simulink model "yixiang"  (R2024a)
settings: Solver=FixedStepDiscrete  StartTime=0.0  StopTime=0.01  FixedStep=1e-8  RelTol=1e-3
libraries: hdlsllib x60, simulink x1
(part 2 of 2)

== system yixiang/CBSVPWM/jxcbsv/yixianga ==
  aH1 : Inport
  zmc1 : Subsystem
  zmcxc6 : Subsystem
  aHyan : Outport
  wires:
  zmcxc6/1(aL1) -> aHyan/1
  zmc1/1(bH1) -> zmcxc6/1(bH1)
  aH1/1 -> zmc1/1(aH1)

== system yixiang/CBSVPWM/jxcbsv/zmc ==
  aH1 : Inport
  Constant2 : Constant  OutDataTypeStr=int16  SampleTime=2E-8
  Constant3 : Constant  Commented=on  Value=0  OutDataTypeStr=int16  SampleTime=2e-8
  Data Type Conversion1 : DataTypeConversion  OutDataTypeStr=boolean  SaturateOnIntegerOverflow=off  RndMeth=Floor
  Data Type Conversion2 : DataTypeConversion  OutDataTypeStr=boolean  SaturateOnIntegerOverflow=off  RndMeth=Floor
  Data Type Conversion3 : DataTypeConversion  Commented=on  OutDataTypeStr=boolean  SaturateOnIntegerOverflow=off  RndMeth=Floor
  HDL Counter1 : hdlsllib/Sources/HDL Counter  Commented=on  CountType=Free running  CountInit=0  CountStep=1  CountMax=250  CountFromType=Initial value  CountFrom=0  CountResetPort=on  CountLoadPort=off  CountEnbPort=off  CountDirPort=off  CountHitOutputPort=off  CountDataType=Signed  CountWordLen=16  CountFracLen=0  CountSampTime=2E-8
  HDL Counter7 : hdlsllib/Sources/HDL Counter  CountType=Free running  CountInit=0  CountStep=1  CountMax=250  CountFromType=Initial value  CountFrom=0  CountResetPort=on  CountLoadPort=off  CountEnbPort=on  CountDirPort=off  CountHitOutputPort=off  CountDataType=Signed  CountWordLen=16  CountFracLen=0  CountSampTime=1
  Logical Operator : Logic  Operator=NOT  AllPortsSameDT=off  OutDataTypeStr=boolean
  Logical Operator1 : Logic  Commented=on  Operator=NOT  AllPortsSameDT=off  OutDataTypeStr=boolean
  Scope6 : Scope  NumInputPorts=2
  Switch : Switch  Threshold=3  SaturateOnIntegerOverflow=off  InputSameDT=off
  Switch2 : Switch  Commented=on  Threshold=1  SaturateOnIntegerOverflow=off  InputSameDT=off
  bH1 : Outport
  wires:
  HDL Counter7/1 -> Switch/2, Scope6/1
  Data Type Conversion1/1 -> Logical Operator/1
  Constant2/1 -> Switch/3
  aH1/1 -> Data Type Conversion1/1, Scope6/2, Data Type Conversion2/1, Switch/1
  Logical Operator/1 -> HDL Counter7/2
  Data Type Conversion2/1 -> HDL Counter7/1
  Constant3/1 -> Switch2/3
  HDL Counter1/1 -> Switch2/2
  Switch/1 -> bH1/1
  Data Type Conversion3/1 -> Logical Operator1/1
  Logical Operator1/1 -> HDL Counter1/1

== system yixiang/CBSVPWM/jxcbsv/zmc1 ==
  aH1 : Inport
  Constant2 : Constant  OutDataTypeStr=int16  SampleTime=2E-8
  Constant3 : Constant  Commented=on  Value=0  OutDataTypeStr=int16  SampleTime=2e-8
  Data Type Conversion1 : DataTypeConversion  OutDataTypeStr=boolean  SaturateOnIntegerOverflow=off  RndMeth=Floor
  Data Type Conversion2 : DataTypeConversion  OutDataTypeStr=boolean  SaturateOnIntegerOverflow=off  RndMeth=Floor
  Data Type Conversion3 : DataTypeConversion  Commented=on  OutDataTypeStr=boolean  SaturateOnIntegerOverflow=off  RndMeth=Floor
  HDL Counter1 : hdlsllib/Sources/HDL Counter  Commented=on  CountType=Free running  CountInit=0  CountStep=1  CountMax=250  CountFromType=Initial value  CountFrom=0  CountResetPort=on  CountLoadPort=off  CountEnbPort=off  CountDirPort=off  CountHitOutputPort=off  CountDataType=Signed  CountWordLen=16  CountFracLen=0  CountSampTime=2E-8
  HDL Counter7 : hdlsllib/Sources/HDL Counter  CountType=Free running  CountInit=0  CountStep=1  CountMax=250  CountFromType=Initial value  CountFrom=0  CountResetPort=on  CountLoadPort=off  CountEnbPort=on  CountDirPort=off  CountHitOutputPort=off  CountDataType=Signed  CountWordLen=16  CountFracLen=0  CountSampTime=1
  Logical Operator : Logic  Operator=NOT  AllPortsSameDT=off  OutDataTypeStr=boolean
  Logical Operator1 : Logic  Commented=on  Operator=NOT  AllPortsSameDT=off  OutDataTypeStr=boolean
  Scope6 : Scope  NumInputPorts=2
  Switch : Switch  Threshold=3  SaturateOnIntegerOverflow=off  InputSameDT=off
  Switch2 : Switch  Commented=on  Threshold=1  SaturateOnIntegerOverflow=off  InputSameDT=off
  bH1 : Outport
  wires:
  HDL Counter7/1 -> Switch/2, Scope6/1
  Data Type Conversion1/1 -> Logical Operator/1
  Constant2/1 -> Switch/3
  aH1/1 -> Data Type Conversion1/1, Scope6/2, Data Type Conversion2/1, Switch/1
  Logical Operator/1 -> HDL Counter7/2
  Data Type Conversion2/1 -> HDL Counter7/1
  Constant3/1 -> Switch2/3
  HDL Counter1/1 -> Switch2/2
  Switch/1 -> bH1/1
  Data Type Conversion3/1 -> Logical Operator1/1
  Logical Operator1/1 -> HDL Counter1/1

== system yixiang/CBSVPWM/jxcbsv/zmc10 ==
  aH1 : Inport
  Constant2 : Constant  OutDataTypeStr=int16  SampleTime=2E-8
  Constant3 : Constant  Commented=on  Value=0  OutDataTypeStr=int16  SampleTime=2e-8
  Data Type Conversion1 : DataTypeConversion  OutDataTypeStr=boolean  SaturateOnIntegerOverflow=off  RndMeth=Floor
  Data Type Conversion2 : DataTypeConversion  OutDataTypeStr=boolean  SaturateOnIntegerOverflow=off  RndMeth=Floor
  Data Type Conversion3 : DataTypeConversion  Commented=on  OutDataTypeStr=boolean  SaturateOnIntegerOverflow=off  RndMeth=Floor
  HDL Counter1 : hdlsllib/Sources/HDL Counter  Commented=on  CountType=Free running  CountInit=0  CountStep=1  CountMax=250  CountFromType=Initial value  CountFrom=0  CountResetPort=on  CountLoadPort=off  CountEnbPort=off  CountDirPort=off  CountHitOutputPort=off  CountDataType=Signed  CountWordLen=16  CountFracLen=0  CountSampTime=2E-8
  HDL Counter7 : hdlsllib/Sources/HDL Counter  CountType=Free running  CountInit=0  CountStep=1  CountMax=250  CountFromType=Initial value  CountFrom=0  CountResetPort=on  CountLoadPort=off  CountEnbPort=on  CountDirPort=off  CountHitOutputPort=off  CountDataType=Signed  CountWordLen=16  CountFracLen=0  CountSampTime=1
  Logical Operator : Logic  Operator=NOT  AllPortsSameDT=off  OutDataTypeStr=boolean
  Logical Operator1 : Logic  Commented=on  Operator=NOT  AllPortsSameDT=off  OutDataTypeStr=boolean
  Scope6 : Scope  NumInputPorts=2
  Switch : Switch  Threshold=3  SaturateOnIntegerOverflow=off  InputSameDT=off
  Switch2 : Switch  Commented=on  Threshold=1  SaturateOnIntegerOverflow=off  InputSameDT=off
  bH1 : Outport
  wires:
  HDL Counter7/1 -> Switch/2, Scope6/1
  Data Type Conversion1/1 -> Logical Operator/1
  Constant2/1 -> Switch/3
  aH1/1 -> Data Type Conversion1/1, Scope6/2, Data Type Conversion2/1, Switch/1
  Logical Operator/1 -> HDL Counter7/2
  Data Type Conversion2/1 -> HDL Counter7/1
  Constant3/1 -> Switch2/3
  HDL Counter1/1 -> Switch2/2
  Switch/1 -> bH1/1
  Data Type Conversion3/1 -> Logical Operator1/1
  Logical Operator1/1 -> HDL Counter1/1

== system yixiang/CBSVPWM/jxcbsv/zmc11 ==
  aH1 : Inport
  Constant2 : Constant  OutDataTypeStr=int16  SampleTime=2E-8
  Constant3 : Constant  Commented=on  Value=0  OutDataTypeStr=int16  SampleTime=2e-8
  Data Type Conversion1 : DataTypeConversion  OutDataTypeStr=boolean  SaturateOnIntegerOverflow=off  RndMeth=Floor
  Data Type Conversion2 : DataTypeConversion  OutDataTypeStr=boolean  SaturateOnIntegerOverflow=off  RndMeth=Floor
  Data Type Conversion3 : DataTypeConversion  Commented=on  OutDataTypeStr=boolean  SaturateOnIntegerOverflow=off  RndMeth=Floor
  HDL Counter1 : hdlsllib/Sources/HDL Counter  Commented=on  CountType=Free running  CountInit=0  CountStep=1  CountMax=250  CountFromType=Initial value  CountFrom=0  CountResetPort=on  CountLoadPort=off  CountEnbPort=off  CountDirPort=off  CountHitOutputPort=off  CountDataType=Signed  CountWordLen=16  CountFracLen=0  CountSampTime=2E-8
  HDL Counter7 : hdlsllib/Sources/HDL Counter  CountType=Free running  CountInit=0  CountStep=1  CountMax=250  CountFromType=Initial value  CountFrom=0  CountResetPort=on  CountLoadPort=off  CountEnbPort=on  CountDirPort=off  CountHitOutputPort=off  CountDataType=Signed  CountWordLen=16  CountFracLen=0  CountSampTime=1
  Logical Operator : Logic  Operator=NOT  AllPortsSameDT=off  OutDataTypeStr=boolean
  Logical Operator1 : Logic  Commented=on  Operator=NOT  AllPortsSameDT=off  OutDataTypeStr=boolean
  Scope6 : Scope  NumInputPorts=2
  Switch : Switch  Threshold=3  SaturateOnIntegerOverflow=off  InputSameDT=off
  Switch2 : Switch  Commented=on  Threshold=1  SaturateOnIntegerOverflow=off  InputSameDT=off
  bH1 : Outport
  wires:
  HDL Counter7/1 -> Switch/2, Scope6/1
  Data Type Conversion1/1 -> Logical Operator/1
  Constant2/1 -> Switch/3
  aH1/1 -> Data Type Conversion1/1, Scope6/2, Data Type Conversion2/1, Switch/1
  Logical Operator/1 -> HDL Counter7/2
  Data Type Conversion2/1 -> HDL Counter7/1
  Constant3/1 -> Switch2/3
  HDL Counter1/1 -> Switch2/2
  Switch/1 -> bH1/1
  Data Type Conversion3/1 -> Logical Operator1/1
  Logical Operator1/1 -> HDL Counter1/1

== system yixiang/CBSVPWM/jxcbsv/zmc2 ==
  aH1 : Inport
  Constant2 : Constant  OutDataTypeStr=int16  SampleTime=2E-8
  Constant3 : Constant  Commented=on  Value=0  OutDataTypeStr=int16  SampleTime=2e-8
  Data Type Conversion1 : DataTypeConversion  OutDataTypeStr=boolean  SaturateOnIntegerOverflow=off  RndMeth=Floor
  Data Type Conversion2 : DataTypeConversion  OutDataTypeStr=boolean  SaturateOnIntegerOverflow=off  RndMeth=Floor
  Data Type Conversion3 : DataTypeConversion  Commented=on  OutDataTypeStr=boolean  SaturateOnIntegerOverflow=off  RndMeth=Floor
  HDL Counter1 : hdlsllib/Sources/HDL Counter  Commented=on  CountType=Free running  CountInit=0  CountStep=1  CountMax=250  CountFromType=Initial value  CountFrom=0  CountResetPort=on  CountLoadPort=off  CountEnbPort=off  CountDirPort=off  CountHitOutputPort=off  CountDataType=Signed  CountWordLen=16  CountFracLen=0  CountSampTime=2E-8
  HDL Counter7 : hdlsllib/Sources/HDL Counter  CountType=Free running  CountInit=0  CountStep=1  CountMax=250  CountFromType=Initial value  CountFrom=0  CountResetPort=on  CountLoadPort=off  CountEnbPort=on  CountDirPort=off  CountHitOutputPort=off  CountDataType=Signed  CountWordLen=16  CountFracLen=0  CountSampTime=1
  Logical Operator : Logic  Operator=NOT  AllPortsSameDT=off  OutDataTypeStr=boolean
  Logical Operator1 : Logic  Commented=on  Operator=NOT  AllPortsSameDT=off  OutDataTypeStr=boolean
  Scope6 : Scope  NumInputPorts=2
  Switch : Switch  Threshold=3  SaturateOnIntegerOverflow=off  InputSameDT=off
  Switch2 : Switch  Commented=on  Threshold=1  SaturateOnIntegerOverflow=off  InputSameDT=off
  bH1 : Outport
  wires:
  HDL Counter7/1 -> Switch/2, Scope6/1
  Data Type Conversion1/1 -> Logical Operator/1
  Constant2/1 -> Switch/3
  aH1/1 -> Data Type Conversion1/1, Scope6/2, Data Type Conversion2/1, Switch/1
  Logical Operator/1 -> HDL Counter7/2
  Data Type Conversion2/1 -> HDL Counter7/1
  Constant3/1 -> Switch2/3
  HDL Counter1/1 -> Switch2/2
  Switch/1 -> bH1/1
  Data Type Conversion3/1 -> Logical Operator1/1
  Logical Operator1/1 -> HDL Counter1/1

== system yixiang/CBSVPWM/jxcbsv/zmc3 ==
  aH1 : Inport
  Constant2 : Constant  OutDataTypeStr=int16  SampleTime=2E-8
  Constant3 : Constant  Commented=on  Value=0  OutDataTypeStr=int16  SampleTime=2e-8
  Data Type Conversion1 : DataTypeConversion  OutDataTypeStr=boolean  SaturateOnIntegerOverflow=off  RndMeth=Floor
  Data Type Conversion2 : DataTypeConversion  OutDataTypeStr=boolean  SaturateOnIntegerOverflow=off  RndMeth=Floor
  Data Type Conversion3 : DataTypeConversion  Commented=on  OutDataTypeStr=boolean  SaturateOnIntegerOverflow=off  RndMeth=Floor
  HDL Counter1 : hdlsllib/Sources/HDL Counter  Commented=on  CountType=Free running  CountInit=0  CountStep=1  CountMax=250  CountFromType=Initial value  CountFrom=0  CountResetPort=on  CountLoadPort=off  CountEnbPort=off  CountDirPort=off  CountHitOutputPort=off  CountDataType=Signed  CountWordLen=16  CountFracLen=0  CountSampTime=2E-8
  HDL Counter7 : hdlsllib/Sources/HDL Counter  CountType=Free running  CountInit=0  CountStep=1  CountMax=250  CountFromType=Initial value  CountFrom=0  CountResetPort=on  CountLoadPort=off  CountEnbPort=on  CountDirPort=off  CountHitOutputPort=off  CountDataType=Signed  CountWordLen=16  CountFracLen=0  CountSampTime=1
  Logical Operator : Logic  Operator=NOT  AllPortsSameDT=off  OutDataTypeStr=boolean
  Logical Operator1 : Logic  Commented=on  Operator=NOT  AllPortsSameDT=off  OutDataTypeStr=boolean
  Scope6 : Scope  NumInputPorts=2
  Switch : Switch  Threshold=3  SaturateOnIntegerOverflow=off  InputSameDT=off
  Switch2 : Switch  Commented=on  Threshold=1  SaturateOnIntegerOverflow=off  InputSameDT=off
  bH1 : Outport
  wires:
  HDL Counter7/1 -> Switch/2, Scope6/1
  Data Type Conversion1/1 -> Logical Operator/1
  Constant2/1 -> Switch/3
  aH1/1 -> Data Type Conversion1/1, Scope6/2, Data Type Conversion2/1, Switch/1
  Logical Operator/1 -> HDL Counter7/2
  Data Type Conversion2/1 -> HDL Counter7/1
  Constant3/1 -> Switch2/3
  HDL Counter1/1 -> Switch2/2
  Switch/1 -> bH1/1
  Data Type Conversion3/1 -> Logical Operator1/1
  Logical Operator1/1 -> HDL Counter1/1

== system yixiang/CBSVPWM/jxcbsv/zmc4 ==
  aH1 : Inport
  Constant2 : Constant  OutDataTypeStr=int16  SampleTime=2E-8
  Constant3 : Constant  Commented=on  Value=0  OutDataTypeStr=int16  SampleTime=2e-8
  Data Type Conversion1 : DataTypeConversion  OutDataTypeStr=boolean  SaturateOnIntegerOverflow=off  RndMeth=Floor
  Data Type Conversion2 : DataTypeConversion  OutDataTypeStr=boolean  SaturateOnIntegerOverflow=off  RndMeth=Floor
  Data Type Conversion3 : DataTypeConversion  Commented=on  OutDataTypeStr=boolean  SaturateOnIntegerOverflow=off  RndMeth=Floor
  HDL Counter1 : hdlsllib/Sources/HDL Counter  Commented=on  CountType=Free running  CountInit=0  CountStep=1  CountMax=250  CountFromType=Initial value  CountFrom=0  CountResetPort=on  CountLoadPort=off  CountEnbPort=off  CountDirPort=off  CountHitOutputPort=off  CountDataType=Signed  CountWordLen=16  CountFracLen=0  CountSampTime=2E-8
  HDL Counter7 : hdlsllib/Sources/HDL Counter  CountType=Free running  CountInit=0  CountStep=1  CountMax=250  CountFromType=Initial value  CountFrom=0  CountResetPort=on  CountLoadPort=off  CountEnbPort=on  CountDirPort=off  CountHitOutputPort=off  CountDataType=Signed  CountWordLen=16  CountFracLen=0  CountSampTime=1
  Logical Operator : Logic  Operator=NOT  AllPortsSameDT=off  OutDataTypeStr=boolean
  Logical Operator1 : Logic  Commented=on  Operator=NOT  AllPortsSameDT=off  OutDataTypeStr=boolean
  Scope6 : Scope  NumInputPorts=2
  Switch : Switch  Threshold=3  SaturateOnIntegerOverflow=off  InputSameDT=off
  Switch2 : Switch  Commented=on  Threshold=1  SaturateOnIntegerOverflow=off  InputSameDT=off
  bH1 : Outport
  wires:
  HDL Counter7/1 -> Switch/2, Scope6/1
  Data Type Conversion1/1 -> Logical Operator/1
  Constant2/1 -> Switch/3
  aH1/1 -> Data Type Conversion1/1, Scope6/2, Data Type Conversion2/1, Switch/1
  Logical Operator/1 -> HDL Counter7/2
  Data Type Conversion2/1 -> HDL Counter7/1
  Constant3/1 -> Switch2/3
  HDL Counter1/1 -> Switch2/2
  Switch/1 -> bH1/1
  Data Type Conversion3/1 -> Logical Operator1/1
  Logical Operator1/1 -> HDL Counter1/1

== system yixiang/CBSVPWM/jxcbsv/zmc5 ==
  aH1 : Inport
  Constant2 : Constant  OutDataTypeStr=int16  SampleTime=2E-8
  Constant3 : Constant  Commented=on  Value=0  OutDataTypeStr=int16  SampleTime=2e-8
  Data Type Conversion1 : DataTypeConversion  OutDataTypeStr=boolean  SaturateOnIntegerOverflow=off  RndMeth=Floor
  Data Type Conversion2 : DataTypeConversion  OutDataTypeStr=boolean  SaturateOnIntegerOverflow=off  RndMeth=Floor
  Data Type Conversion3 : DataTypeConversion  Commented=on  OutDataTypeStr=boolean  SaturateOnIntegerOverflow=off  RndMeth=Floor
  HDL Counter1 : hdlsllib/Sources/HDL Counter  Commented=on  CountType=Free running  CountInit=0  CountStep=1  CountMax=250  CountFromType=Initial value  CountFrom=0  CountResetPort=on  CountLoadPort=off  CountEnbPort=off  CountDirPort=off  CountHitOutputPort=off  CountDataType=Signed  CountWordLen=16  CountFracLen=0  CountSampTime=2E-8
  HDL Counter7 : hdlsllib/Sources/HDL Counter  CountType=Free running  CountInit=0  CountStep=1  CountMax=250  CountFromType=Initial value  CountFrom=0  CountResetPort=on  CountLoadPort=off  CountEnbPort=on  CountDirPort=off  CountHitOutputPort=off  CountDataType=Signed  CountWordLen=16  CountFracLen=0  CountSampTime=1
  Logical Operator : Logic  Operator=NOT  AllPortsSameDT=off  OutDataTypeStr=boolean
  Logical Operator1 : Logic  Commented=on  Operator=NOT  AllPortsSameDT=off  OutDataTypeStr=boolean
  Scope6 : Scope  NumInputPorts=2
  Switch : Switch  Threshold=3  SaturateOnIntegerOverflow=off  InputSameDT=off
  Switch2 : Switch  Commented=on  Threshold=1  SaturateOnIntegerOverflow=off  InputSameDT=off
  bH1 : Outport
  wires:
  HDL Counter7/1 -> Switch/2, Scope6/1
  Data Type Conversion1/1 -> Logical Operator/1
  Constant2/1 -> Switch/3
  aH1/1 -> Data Type Conversion1/1, Scope6/2, Data Type Conversion2/1, Switch/1
  Logical Operator/1 -> HDL Counter7/2
  Data Type Conversion2/1 -> HDL Counter7/1
  Constant3/1 -> Switch2/3
  HDL Counter1/1 -> Switch2/2
  Switch/1 -> bH1/1
  Data Type Conversion3/1 -> Logical Operator1/1
  Logical Operator1/1 -> HDL Counter1/1

== system yixiang/CBSVPWM/jxcbsv/zmc6 ==
  aH1 : Inport
  Constant2 : Constant  OutDataTypeStr=int16  SampleTime=2E-8
  Constant3 : Constant  Commented=on  Value=0  OutDataTypeStr=int16  SampleTime=2e-8
  Data Type Conversion1 : DataTypeConversion  OutDataTypeStr=boolean  SaturateOnIntegerOverflow=off  RndMeth=Floor
  Data Type Conversion2 : DataTypeConversion  OutDataTypeStr=boolean  SaturateOnIntegerOverflow=off  RndMeth=Floor
  Data Type Conversion3 : DataTypeConversion  Commented=on  OutDataTypeStr=boolean  SaturateOnIntegerOverflow=off  RndMeth=Floor
  HDL Counter1 : hdlsllib/Sources/HDL Counter  Commented=on  CountType=Free running  CountInit=0  CountStep=1  CountMax=250  CountFromType=Initial value  CountFrom=0  CountResetPort=on  CountLoadPort=off  CountEnbPort=off  CountDirPort=off  CountHitOutputPort=off  CountDataType=Signed  CountWordLen=16  CountFracLen=0  CountSampTime=2E-8
  HDL Counter7 : hdlsllib/Sources/HDL Counter  CountType=Free running  CountInit=0  CountStep=1  CountMax=250  CountFromType=Initial value  CountFrom=0  CountResetPort=on  CountLoadPort=off  CountEnbPort=on  CountDirPort=off  CountHitOutputPort=off  CountDataType=Signed  CountWordLen=16  CountFracLen=0  CountSampTime=1
  Logical Operator : Logic  Operator=NOT  AllPortsSameDT=off  OutDataTypeStr=boolean
  Logical Operator1 : Logic  Commented=on  Operator=NOT  AllPortsSameDT=off  OutDataTypeStr=boolean
  Scope6 : Scope  NumInputPorts=2
  Switch : Switch  Threshold=3  SaturateOnIntegerOverflow=off  InputSameDT=off
  Switch2 : Switch  Commented=on  Threshold=1  SaturateOnIntegerOverflow=off  InputSameDT=off
  bH1 : Outport
  wires:
  HDL Counter7/1 -> Switch/2, Scope6/1
  Data Type Conversion1/1 -> Logical Operator/1
  Constant2/1 -> Switch/3
  aH1/1 -> Data Type Conversion1/1, Scope6/2, Data Type Conversion2/1, Switch/1
  Logical Operator/1 -> HDL Counter7/2
  Data Type Conversion2/1 -> HDL Counter7/1
  Constant3/1 -> Switch2/3
  HDL Counter1/1 -> Switch2/2
  Switch/1 -> bH1/1
  Data Type Conversion3/1 -> Logical Operator1/1
  Logical Operator1/1 -> HDL Counter1/1

== system yixiang/CBSVPWM/jxcbsv/zmc7 ==
  aH1 : Inport
  Constant2 : Constant  OutDataTypeStr=int16  SampleTime=2E-8
  Constant3 : Constant  Commented=on  Value=0  OutDataTypeStr=int16  SampleTime=2e-8
  Data Type Conversion1 : DataTypeConversion  OutDataTypeStr=boolean  SaturateOnIntegerOverflow=off  RndMeth=Floor
  Data Type Conversion2 : DataTypeConversion  OutDataTypeStr=boolean  SaturateOnIntegerOverflow=off  RndMeth=Floor
  Data Type Conversion3 : DataTypeConversion  Commented=on  OutDataTypeStr=boolean  SaturateOnIntegerOverflow=off  RndMeth=Floor
  HDL Counter1 : hdlsllib/Sources/HDL Counter  Commented=on  CountType=Free running  CountInit=0  CountStep=1  CountMax=250  CountFromType=Initial value  CountFrom=0  CountResetPort=on  CountLoadPort=off  CountEnbPort=off  CountDirPort=off  CountHitOutputPort=off  CountDataType=Signed  CountWordLen=16  CountFracLen=0  CountSampTime=2E-8
  HDL Counter7 : hdlsllib/Sources/HDL Counter  CountType=Free running  CountInit=0  CountStep=1  CountMax=250  CountFromType=Initial value  CountFrom=0  CountResetPort=on  CountLoadPort=off  CountEnbPort=on  CountDirPort=off  CountHitOutputPort=off  CountDataType=Signed  CountWordLen=16  CountFracLen=0  CountSampTime=1
  Logical Operator : Logic  Operator=NOT  AllPortsSameDT=off  OutDataTypeStr=boolean
  Logical Operator1 : Logic  Commented=on  Operator=NOT  AllPortsSameDT=off  OutDataTypeStr=boolean
  Scope6 : Scope  NumInputPorts=2
  Switch : Switch  Threshold=3  SaturateOnIntegerOverflow=off  InputSameDT=off
  Switch2 : Switch  Commented=on  Threshold=1  SaturateOnIntegerOverflow=off  InputSameDT=off
  bH1 : Outport
  wires:
  HDL Counter7/1 -> Switch/2, Scope6/1
  Data Type Conversion1/1 -> Logical Operator/1
  Constant2/1 -> Switch/3
  aH1/1 -> Data Type Conversion1/1, Scope6/2, Data Type Conversion2/1, Switch/1
  Logical Operator/1 -> HDL Counter7/2
  Data Type Conversion2/1 -> HDL Counter7/1
  Constant3/1 -> Switch2/3
  HDL Counter1/1 -> Switch2/2
  Switch/1 -> bH1/1
  Data Type Conversion3/1 -> Logical Operator1/1
  Logical Operator1/1 -> HDL Counter1/1

== system yixiang/CBSVPWM/jxcbsv/zmc8 ==
  aH1 : Inport
  Constant2 : Constant  OutDataTypeStr=int16  SampleTime=2E-8
  Constant3 : Constant  Commented=on  Value=0  OutDataTypeStr=int16  SampleTime=2e-8
  Data Type Conversion1 : DataTypeConversion  OutDataTypeStr=boolean  SaturateOnIntegerOverflow=off  RndMeth=Floor
  Data Type Conversion2 : DataTypeConversion  OutDataTypeStr=boolean  SaturateOnIntegerOverflow=off  RndMeth=Floor
  Data Type Conversion3 : DataTypeConversion  Commented=on  OutDataTypeStr=boolean  SaturateOnIntegerOverflow=off  RndMeth=Floor
  HDL Counter1 : hdlsllib/Sources/HDL Counter  Commented=on  CountType=Free running  CountInit=0  CountStep=1  CountMax=250  CountFromType=Initial value  CountFrom=0  CountResetPort=on  CountLoadPort=off  CountEnbPort=off  CountDirPort=off  CountHitOutputPort=off  CountDataType=Signed  CountWordLen=16  CountFracLen=0  CountSampTime=2E-8
  HDL Counter7 : hdlsllib/Sources/HDL Counter  CountType=Free running  CountInit=0  CountStep=1  CountMax=250  CountFromType=Initial value  CountFrom=0  CountResetPort=on  CountLoadPort=off  CountEnbPort=on  CountDirPort=off  CountHitOutputPort=off  CountDataType=Signed  CountWordLen=16  CountFracLen=0  CountSampTime=1
  Logical Operator : Logic  Operator=NOT  AllPortsSameDT=off  OutDataTypeStr=boolean
  Logical Operator1 : Logic  Commented=on  Operator=NOT  AllPortsSameDT=off  OutDataTypeStr=boolean
  Scope6 : Scope  NumInputPorts=2
  Switch : Switch  Threshold=3  SaturateOnIntegerOverflow=off  InputSameDT=off
  Switch2 : Switch  Commented=on  Threshold=1  SaturateOnIntegerOverflow=off  InputSameDT=off
  bH1 : Outport
  wires:
  HDL Counter7/1 -> Switch/2, Scope6/1
  Data Type Conversion1/1 -> Logical Operator/1
  Constant2/1 -> Switch/3
  aH1/1 -> Data Type Conversion1/1, Scope6/2, Data Type Conversion2/1, Switch/1
  Logical Operator/1 -> HDL Counter7/2
  Data Type Conversion2/1 -> HDL Counter7/1
  Constant3/1 -> Switch2/3
  HDL Counter1/1 -> Switch2/2
  Switch/1 -> bH1/1
  Data Type Conversion3/1 -> Logical Operator1/1
  Logical Operator1/1 -> HDL Counter1/1

== system yixiang/CBSVPWM/jxcbsv/zmc9 ==
  aH1 : Inport
  Constant2 : Constant  OutDataTypeStr=int16  SampleTime=2E-8
  Constant3 : Constant  Commented=on  Value=0  OutDataTypeStr=int16  SampleTime=2e-8
  Data Type Conversion1 : DataTypeConversion  OutDataTypeStr=boolean  SaturateOnIntegerOverflow=off  RndMeth=Floor
  Data Type Conversion2 : DataTypeConversion  OutDataTypeStr=boolean  SaturateOnIntegerOverflow=off  RndMeth=Floor
  Data Type Conversion3 : DataTypeConversion  Commented=on  OutDataTypeStr=boolean  SaturateOnIntegerOverflow=off  RndMeth=Floor
  HDL Counter1 : hdlsllib/Sources/HDL Counter  Commented=on  CountType=Free running  CountInit=0  CountStep=1  CountMax=250  CountFromType=Initial value  CountFrom=0  CountResetPort=on  CountLoadPort=off  CountEnbPort=off  CountDirPort=off  CountHitOutputPort=off  CountDataType=Signed  CountWordLen=16  CountFracLen=0  CountSampTime=2E-8
  HDL Counter7 : hdlsllib/Sources/HDL Counter  CountType=Free running  CountInit=0  CountStep=1  CountMax=250  CountFromType=Initial value  CountFrom=0  CountResetPort=on  CountLoadPort=off  CountEnbPort=on  CountDirPort=off  CountHitOutputPort=off  CountDataType=Signed  CountWordLen=16  CountFracLen=0  CountSampTime=1
  Logical Operator : Logic  Operator=NOT  AllPortsSameDT=off  OutDataTypeStr=boolean
  Logical Operator1 : Logic  Commented=on  Operator=NOT  AllPortsSameDT=off  OutDataTypeStr=boolean
  Scope6 : Scope  NumInputPorts=2
  Switch : Switch  Threshold=3  SaturateOnIntegerOverflow=off  InputSameDT=off
  Switch2 : Switch  Commented=on  Threshold=1  SaturateOnIntegerOverflow=off  InputSameDT=off
  bH1 : Outport
  wires:
  HDL Counter7/1 -> Switch/2, Scope6/1
  Data Type Conversion1/1 -> Logical Operator/1
  Constant2/1 -> Switch/3
  aH1/1 -> Data Type Conversion1/1, Scope6/2, Data Type Conversion2/1, Switch/1
  Logical Operator/1 -> HDL Counter7/2
  Data Type Conversion2/1 -> HDL Counter7/1
  Constant3/1 -> Switch2/3
  HDL Counter1/1 -> Switch2/2
  Switch/1 -> bH1/1
  Data Type Conversion3/1 -> Logical Operator1/1
  Logical Operator1/1 -> HDL Counter1/1

== system yixiang/CBSVPWM/jxcbsv/zmcxc ==
  bH1 : Inport
  Constant2 : Constant  Value=0  OutDataTypeStr=int16  SampleTime=2e-8
  Data Type Conversion3 : DataTypeConversion  OutDataTypeStr=boolean  SaturateOnIntegerOverflow=off  RndMeth=Floor
  Data Type Conversion4 : DataTypeConversion  OutDataTypeStr=boolean  SaturateOnIntegerOverflow=off  RndMeth=Floor
  Logical Operator2 : Logic  Operator=NOT  AllPortsSameDT=off  OutDataTypeStr=boolean
  Switch3 : Switch  Threshold=6  SaturateOnIntegerOverflow=off  InputSameDT=off
  高电平计数 : hdlsllib/Sources/HDL Counter  CountType=Free running  CountInit=0  CountStep=1  CountMax=250  CountFromType=Initial value  CountFrom=0  CountResetPort=on  CountLoadPort=off  CountEnbPort=on  CountDirPort=off  CountHitOutputPort=off  CountDataType=Signed  CountWordLen=16  CountFracLen=0  CountSampTime=1
  aL1 : Outport
  wires:
  Data Type Conversion3/1 -> Logical Operator2/1
  bH1/1 -> Switch3/1, Data Type Conversion4/1, Data Type Conversion3/1
  Constant2/1 -> Switch3/3
  高电平计数/1 -> Switch3/2
  Logical Operator2/1 -> 高电平计数/1
  Data Type Conversion4/1 -> 高电平计数/2
  Switch3/1 -> aL1/1

== system yixiang/CBSVPWM/jxcbsv/zmcxc1 ==
  bH1 : Inport
  Constant2 : Constant  Value=0  OutDataTypeStr=int16  SampleTime=2e-8
  Data Type Conversion3 : DataTypeConversion  OutDataTypeStr=boolean  SaturateOnIntegerOverflow=off  RndMeth=Floor
  Data Type Conversion4 : DataTypeConversion  OutDataTypeStr=boolean  SaturateOnIntegerOverflow=off  RndMeth=Floor
  Logical Operator2 : Logic  Operator=NOT  AllPortsSameDT=off  OutDataTypeStr=boolean
  Switch3 : Switch  Threshold=6  SaturateOnIntegerOverflow=off  InputSameDT=off
  高电平计数 : hdlsllib/Sources/HDL Counter  CountType=Free running  CountInit=0  CountStep=1  CountMax=250  CountFromType=Initial value  CountFrom=0  CountResetPort=on  CountLoadPort=off  CountEnbPort=on  CountDirPort=off  CountHitOutputPort=off  CountDataType=Signed  CountWordLen=16  CountFracLen=0  CountSampTime=1
  aL1 : Outport
  wires:
  Data Type Conversion3/1 -> Logical Operator2/1
  bH1/1 -> Switch3/1, Data Type Conversion4/1, Data Type Conversion3/1
  Constant2/1 -> Switch3/3
  高电平计数/1 -> Switch3/2
  Logical Operator2/1 -> 高电平计数/1
  Data Type Conversion4/1 -> 高电平计数/2
  Switch3/1 -> aL1/1

== system yixiang/CBSVPWM/jxcbsv/zmcxc2 ==
  bH1 : Inport
  Constant2 : Constant  Value=0  OutDataTypeStr=int16  SampleTime=2e-8
  Data Type Conversion3 : DataTypeConversion  OutDataTypeStr=boolean  SaturateOnIntegerOverflow=off  RndMeth=Floor
  Data Type Conversion4 : DataTypeConversion  OutDataTypeStr=boolean  SaturateOnIntegerOverflow=off  RndMeth=Floor
  Logical Operator2 : Logic  Operator=NOT  AllPortsSameDT=off  OutDataTypeStr=boolean
  Switch3 : Switch  Threshold=6  SaturateOnIntegerOverflow=off  InputSameDT=off
  高电平计数 : hdlsllib/Sources/HDL Counter  CountType=Free running  CountInit=0  CountStep=1  CountMax=250  CountFromType=Initial value  CountFrom=0  CountResetPort=on  CountLoadPort=off  CountEnbPort=on  CountDirPort=off  CountHitOutputPort=off  CountDataType=Signed  CountWordLen=16  CountFracLen=0  CountSampTime=1
  aL1 : Outport
  wires:
  Data Type Conversion3/1 -> Logical Operator2/1
  bH1/1 -> Switch3/1, Data Type Conversion4/1, Data Type Conversion3/1
  Constant2/1 -> Switch3/3
  高电平计数/1 -> Switch3/2
  Logical Operator2/1 -> 高电平计数/1
  Data Type Conversion4/1 -> 高电平计数/2
  Switch3/1 -> aL1/1

== system yixiang/CBSVPWM/jxcbsv/zmcxc3 ==
  bH1 : Inport
  Constant2 : Constant  Value=0  OutDataTypeStr=int16  SampleTime=2e-8
  Data Type Conversion3 : DataTypeConversion  OutDataTypeStr=boolean  SaturateOnIntegerOverflow=off  RndMeth=Floor
  Data Type Conversion4 : DataTypeConversion  OutDataTypeStr=boolean  SaturateOnIntegerOverflow=off  RndMeth=Floor
  Logical Operator2 : Logic  Operator=NOT  AllPortsSameDT=off  OutDataTypeStr=boolean
  Switch3 : Switch  Threshold=6  SaturateOnIntegerOverflow=off  InputSameDT=off
  高电平计数 : hdlsllib/Sources/HDL Counter  CountType=Free running  CountInit=0  CountStep=1  CountMax=250  CountFromType=Initial value  CountFrom=0  CountResetPort=on  CountLoadPort=off  CountEnbPort=on  CountDirPort=off  CountHitOutputPort=off  CountDataType=Signed  CountWordLen=16  CountFracLen=0  CountSampTime=1
  aL1 : Outport
  wires:
  Data Type Conversion3/1 -> Logical Operator2/1
  bH1/1 -> Switch3/1, Data Type Conversion4/1, Data Type Conversion3/1
  Constant2/1 -> Switch3/3
  高电平计数/1 -> Switch3/2
  Logical Operator2/1 -> 高电平计数/1
  Data Type Conversion4/1 -> 高电平计数/2
  Switch3/1 -> aL1/1

== system yixiang/CBSVPWM/jxcbsv/zmcxc4 ==
  bH1 : Inport
  Constant2 : Constant  Value=0  OutDataTypeStr=int16  SampleTime=2e-8
  Data Type Conversion3 : DataTypeConversion  OutDataTypeStr=boolean  SaturateOnIntegerOverflow=off  RndMeth=Floor
  Data Type Conversion4 : DataTypeConversion  OutDataTypeStr=boolean  SaturateOnIntegerOverflow=off  RndMeth=Floor
  Logical Operator2 : Logic  Operator=NOT  AllPortsSameDT=off  OutDataTypeStr=boolean
  Switch3 : Switch  Threshold=6  SaturateOnIntegerOverflow=off  InputSameDT=off
  高电平计数 : hdlsllib/Sources/HDL Counter  CountType=Free running  CountInit=0  CountStep=1  CountMax=250  CountFromType=Initial value  CountFrom=0  CountResetPort=on  CountLoadPort=off  CountEnbPort=on  CountDirPort=off  CountHitOutputPort=off  CountDataType=Signed  CountWordLen=16  CountFracLen=0  CountSampTime=1
  aL1 : Outport
  wires:
  Data Type Conversion3/1 -> Logical Operator2/1
  bH1/1 -> Switch3/1, Data Type Conversion4/1, Data Type Conversion3/1
  Constant2/1 -> Switch3/3
  高电平计数/1 -> Switch3/2
  Logical Operator2/1 -> 高电平计数/1
  Data Type Conversion4/1 -> 高电平计数/2
  Switch3/1 -> aL1/1

== system yixiang/CBSVPWM/jxcbsv/zmcxc5 ==
  bH1 : Inport
  Constant2 : Constant  Value=0  OutDataTypeStr=int16  SampleTime=2e-8
  Data Type Conversion3 : DataTypeConversion  OutDataTypeStr=boolean  SaturateOnIntegerOverflow=off  RndMeth=Floor
  Data Type Conversion4 : DataTypeConversion  OutDataTypeStr=boolean  SaturateOnIntegerOverflow=off  RndMeth=Floor
  Logical Operator2 : Logic  Operator=NOT  AllPortsSameDT=off  OutDataTypeStr=boolean
  Switch3 : Switch  Threshold=6  SaturateOnIntegerOverflow=off  InputSameDT=off
  高电平计数 : hdlsllib/Sources/HDL Counter  CountType=Free running  CountInit=0  CountStep=1  CountMax=250  CountFromType=Initial value  CountFrom=0  CountResetPort=on  CountLoadPort=off  CountEnbPort=on  CountDirPort=off  CountHitOutputPort=off  CountDataType=Signed  CountWordLen=16  CountFracLen=0  CountSampTime=1
  aL1 : Outport
  wires:
  Data Type Conversion3/1 -> Logical Operator2/1
  bH1/1 -> Switch3/1, Data Type Conversion4/1, Data Type Conversion3/1
  Constant2/1 -> Switch3/3
  高电平计数/1 -> Switch3/2
  Logical Operator2/1 -> 高电平计数/1
  Data Type Conversion4/1 -> 高电平计数/2
  Switch3/1 -> aL1/1

== system yixiang/CBSVPWM/jxcbsv/Subsystem/Inverse_Clarke_Transform ==
  Alpha : Inport
  Beta : Inport  Port=2
  Add : Sum  Inputs=-+  OutDataTypeStr=fixdt(1,32,27)
  Add1 : Sum  Inputs=--  OutDataTypeStr=fixdt(1,32,27)
  Data_Type_Convert : DataTypeConversion  OutDataTypeStr=fixdt(1,32,27)  RndMeth=Simplest  SaturateOnIntegerOverflow=off
  Gain : Gain  Gain=1/2  ParamDataTypeStr=fixdt(1,16,15)  OutDataTypeStr=fixdt(1,40,35)
  Gain1 : Gain  Gain=sqrt(3)/2  ParamDataTypeStr=fixdt(1,16,15)  OutDataTypeStr=fixdt(1,40,35)
  Mux : Mux  Inputs=3
  ABC : Outport  VectorParamsAs1DForOutWhenUnconnected=off
  wires:
  Gain/1 -> Add1/1, Add/1
  Gain1/1 -> Add/2, Add1/2
  Add/1 -> Mux/2
  Add1/1 -> Mux/3
  Beta/1 -> Gain1/1
  Alpha/1 -> Gain/1, Data_Type_Convert/1
  Mux/1 -> ABC/1
  Data_Type_Convert/1 -> Mux/1

== system yixiang/CBSVPWM/jxcbsv/Subsystem/Inverse_Park_Transform ==
  D : Inport
  Q : Inport  Port=2
  Sin_Coefficient : Inport  Port=3
  Cos_Coefficient : Inport  Port=4
  Add1 : Sum  Inputs=+-  OutDataTypeStr=fixdt(1,32,27)
  Add2 : Sum  OutDataTypeStr=fixdt(1,32,27)
  Cos_Coefficient1 : InportShadow  Port=4
  Product{1..4} (4 alike) : Product  OutDataTypeStr=fixdt(1,32,27)  RndMeth=Simplest
  Sin_Coefficient1 : InportShadow  Port=3
  Alpha : Outport  VectorParamsAs1DForOutWhenUnconnected=off
  Beta : Outport  Port=2  VectorParamsAs1DForOutWhenUnconnected=off
  wires:
  Add2/1 -> Beta/1
  Add1/1 -> Alpha/1
  Product3/1 -> Add2/1
  Product4/1 -> Add2/2
  Product1/1 -> Add1/1
  Product2/1 -> Add1/2
  Cos_Coefficient1/1 -> Product4/2
  Sin_Coefficient/1 -> Product2/2
  D/1 -> Product3/1, Product1/1
  Q/1 -> Product2/1, Product4/1
  Sin_Coefficient1/1 -> Product3/2
  Cos_Coefficient/1 -> Product1/2

== system yixiang/CBSVPWM/jxcbsv/dqabc/Inverse_Clarke_Transform ==
  Alpha : Inport
  Beta : Inport  Port=2
  Add : Sum  Inputs=-+  OutDataTypeStr=fixdt(1,32,25)
  Add1 : Sum  Inputs=--  OutDataTypeStr=fixdt(1,32,25)
  Data_Type_Convert : DataTypeConversion  OutDataTypeStr=fixdt(1,32,25)  RndMeth=Simplest  SaturateOnIntegerOverflow=off
  Gain : Gain  Gain=1/2  ParamDataTypeStr=fixdt(1,16,15)  OutDataTypeStr=fixdt(1,32,27)
  Gain1 : Gain  Gain=sqrt(3)/2  ParamDataTypeStr=fixdt(1,16,15)  OutDataTypeStr=fixdt(1,32,26)
  Mux : Mux  Inputs=3
  ABC : Outport  VectorParamsAs1DForOutWhenUnconnected=off
  wires:
  Gain/1 -> Add1/1, Add/1
  Gain1/1 -> Add1/2, Add/2
  Add/1 -> Mux/2
  Add1/1 -> Mux/3
  Beta/1 -> Gain1/1
  Alpha/1 -> Gain/1, Data_Type_Convert/1
  Mux/1 -> ABC/1
  Data_Type_Convert/1 -> Mux/1

== system yixiang/CBSVPWM/jxcbsv/dqabc/Inverse_Park_Transform ==
  D : Inport
  Q : Inport  Port=2
  Sin_Coefficient : Inport  Port=3
  Cos_Coefficient : Inport  Port=4
  Add1 : Sum  Inputs=+-  OutDataTypeStr=fixdt(1,32,27)
  Add2 : Sum  OutDataTypeStr=fixdt(1,32,27)
  Cos_Coefficient1 : InportShadow  Port=4
  Product{1..4} (4 alike) : Product  OutDataTypeStr=fixdt(1,32,27)  RndMeth=Simplest
  Sin_Coefficient1 : InportShadow  Port=3
  Alpha : Outport  VectorParamsAs1DForOutWhenUnconnected=off
  Beta : Outport  Port=2  VectorParamsAs1DForOutWhenUnconnected=off
  wires:
  Add2/1 -> Beta/1
  Add1/1 -> Alpha/1
  Product3/1 -> Add2/1
  Product4/1 -> Add2/2
  Product1/1 -> Add1/1
  Product2/1 -> Add1/2
  Cos_Coefficient1/1 -> Product4/2
  Sin_Coefficient/1 -> Product2/2
  D/1 -> Product3/1, Product1/1
  Q/1 -> Product2/1, Product4/1
  Sin_Coefficient1/1 -> Product3/2
  Cos_Coefficient/1 -> Product1/2

== system yixiang/CBSVPWM/jxcbsv/yixiang2/zmc1 ==
  aH1 : Inport
  Constant2 : Constant  OutDataTypeStr=int16  SampleTime=2E-8
  Constant3 : Constant  Commented=on  Value=0  OutDataTypeStr=int16  SampleTime=2e-8
  Data Type Conversion1 : DataTypeConversion  OutDataTypeStr=boolean  SaturateOnIntegerOverflow=off  RndMeth=Floor
  Data Type Conversion2 : DataTypeConversion  OutDataTypeStr=boolean  SaturateOnIntegerOverflow=off  RndMeth=Floor
  Data Type Conversion3 : DataTypeConversion  Commented=on  OutDataTypeStr=boolean  SaturateOnIntegerOverflow=off  RndMeth=Floor
  HDL Counter1 : hdlsllib/Sources/HDL Counter  Commented=on  CountType=Free running  CountInit=0  CountStep=1  CountMax=250  CountFromType=Initial value  CountFrom=0  CountResetPort=on  CountLoadPort=off  CountEnbPort=off  CountDirPort=off  CountHitOutputPort=off  CountDataType=Signed  CountWordLen=16  CountFracLen=0  CountSampTime=2E-8
  HDL Counter7 : hdlsllib/Sources/HDL Counter  CountType=Free running  CountInit=0  CountStep=1  CountMax=250  CountFromType=Initial value  CountFrom=0  CountResetPort=on  CountLoadPort=off  CountEnbPort=on  CountDirPort=off  CountHitOutputPort=off  CountDataType=Signed  CountWordLen=16  CountFracLen=0  CountSampTime=1
  Logical Operator : Logic  Operator=NOT  AllPortsSameDT=off  OutDataTypeStr=boolean
  Logical Operator1 : Logic  Commented=on  Operator=NOT  AllPortsSameDT=off  OutDataTypeStr=boolean
  Scope6 : Scope  NumInputPorts=2
  Switch : Switch  Threshold=3  SaturateOnIntegerOverflow=off  InputSameDT=off
  Switch2 : Switch  Commented=on  Threshold=1  SaturateOnIntegerOverflow=off  InputSameDT=off
  bH1 : Outport
  wires:
  HDL Counter7/1 -> Switch/2, Scope6/1
  Data Type Conversion1/1 -> Logical Operator/1
  Constant2/1 -> Switch/3
  aH1/1 -> Data Type Conversion1/1, Scope6/2, Data Type Conversion2/1, Switch/1
  Logical Operator/1 -> HDL Counter7/2
  Data Type Conversion2/1 -> HDL Counter7/1
  Constant3/1 -> Switch2/3
  HDL Counter1/1 -> Switch2/2
  Switch/1 -> bH1/1
  Data Type Conversion3/1 -> Logical Operator1/1
  Logical Operator1/1 -> HDL Counter1/1

== system yixiang/CBSVPWM/jxcbsv/yixiang2/zmcxc6 ==
  bH1 : Inport
  Constant2 : Constant  Value=0  OutDataTypeStr=int16  SampleTime=2e-8
  Data Type Conversion3 : DataTypeConversion  OutDataTypeStr=boolean  SaturateOnIntegerOverflow=off  RndMeth=Floor
  Data Type Conversion4 : DataTypeConversion  OutDataTypeStr=boolean  SaturateOnIntegerOverflow=off  RndMeth=Floor
  Logical Operator2 : Logic  Operator=NOT  AllPortsSameDT=off  OutDataTypeStr=boolean
  Switch3 : Switch  Threshold=6  SaturateOnIntegerOverflow=off  InputSameDT=off
  高电平计数 : hdlsllib/Sources/HDL Counter  CountType=Free running  CountInit=0  CountStep=1  CountMax=250  CountFromType=Initial value  CountFrom=0  CountResetPort=on  CountLoadPort=off  CountEnbPort=on  CountDirPort=off  CountHitOutputPort=off  CountDataType=Signed  CountWordLen=16  CountFracLen=0  CountSampTime=1
  aL1 : Outport
  wires:
  Data Type Conversion3/1 -> Logical Operator2/1
  bH1/1 -> Switch3/1, Data Type Conversion4/1, Data Type Conversion3/1
  Constant2/1 -> Switch3/3
  高电平计数/1 -> Switch3/2
  Logical Operator2/1 -> 高电平计数/1
  Data Type Conversion4/1 -> 高电平计数/2
  Switch3/1 -> aL1/1

== system yixiang/CBSVPWM/jxcbsv/yixiang4/zmc1 ==
  aH1 : Inport
  Constant2 : Constant  OutDataTypeStr=int16  SampleTime=2E-8
  Constant3 : Constant  Commented=on  Value=0  OutDataTypeStr=int16  SampleTime=2e-8
  Data Type Conversion1 : DataTypeConversion  OutDataTypeStr=boolean  SaturateOnIntegerOverflow=off  RndMeth=Floor
  Data Type Conversion2 : DataTypeConversion  OutDataTypeStr=boolean  SaturateOnIntegerOverflow=off  RndMeth=Floor
  Data Type Conversion3 : DataTypeConversion  Commented=on  OutDataTypeStr=boolean  SaturateOnIntegerOverflow=off  RndMeth=Floor
  HDL Counter1 : hdlsllib/Sources/HDL Counter  Commented=on  CountType=Free running  CountInit=0  CountStep=1  CountMax=250  CountFromType=Initial value  CountFrom=0  CountResetPort=on  CountLoadPort=off  CountEnbPort=off  CountDirPort=off  CountHitOutputPort=off  CountDataType=Signed  CountWordLen=16  CountFracLen=0  CountSampTime=2E-8
  HDL Counter7 : hdlsllib/Sources/HDL Counter  CountType=Free running  CountInit=0  CountStep=1  CountMax=250  CountFromType=Initial value  CountFrom=0  CountResetPort=on  CountLoadPort=off  CountEnbPort=on  CountDirPort=off  CountHitOutputPort=off  CountDataType=Signed  CountWordLen=16  CountFracLen=0  CountSampTime=1
  Logical Operator : Logic  Operator=NOT  AllPortsSameDT=off  OutDataTypeStr=boolean
  Logical Operator1 : Logic  Commented=on  Operator=NOT  AllPortsSameDT=off  OutDataTypeStr=boolean
  Scope6 : Scope  NumInputPorts=2
  Switch : Switch  Threshold=3  SaturateOnIntegerOverflow=off  InputSameDT=off
  Switch2 : Switch  Commented=on  Threshold=1  SaturateOnIntegerOverflow=off  InputSameDT=off
  bH1 : Outport
  wires:
  HDL Counter7/1 -> Switch/2, Scope6/1
  Data Type Conversion1/1 -> Logical Operator/1
  Constant2/1 -> Switch/3
  aH1/1 -> Data Type Conversion1/1, Scope6/2, Data Type Conversion2/1, Switch/1
  Logical Operator/1 -> HDL Counter7/2
  Data Type Conversion2/1 -> HDL Counter7/1
  Constant3/1 -> Switch2/3
  HDL Counter1/1 -> Switch2/2
  Switch/1 -> bH1/1
  Data Type Conversion3/1 -> Logical Operator1/1
  Logical Operator1/1 -> HDL Counter1/1

== system yixiang/CBSVPWM/jxcbsv/yixiang4/zmcxc6 ==
  bH1 : Inport
  Constant2 : Constant  Value=0  OutDataTypeStr=int16  SampleTime=2e-8
  Data Type Conversion3 : DataTypeConversion  OutDataTypeStr=boolean  SaturateOnIntegerOverflow=off  RndMeth=Floor
  Data Type Conversion4 : DataTypeConversion  OutDataTypeStr=boolean  SaturateOnIntegerOverflow=off  RndMeth=Floor
  Logical Operator2 : Logic  Operator=NOT  AllPortsSameDT=off  OutDataTypeStr=boolean
  Switch3 : Switch  Threshold=6  SaturateOnIntegerOverflow=off  InputSameDT=off
  高电平计数 : hdlsllib/Sources/HDL Counter  CountType=Free running  CountInit=0  CountStep=1  CountMax=250  CountFromType=Initial value  CountFrom=0  CountResetPort=on  CountLoadPort=off  CountEnbPort=on  CountDirPort=off  CountHitOutputPort=off  CountDataType=Signed  CountWordLen=16  CountFracLen=0  CountSampTime=1
  aL1 : Outport
  wires:
  Data Type Conversion3/1 -> Logical Operator2/1
  bH1/1 -> Switch3/1, Data Type Conversion4/1, Data Type Conversion3/1
  Constant2/1 -> Switch3/3
  高电平计数/1 -> Switch3/2
  Logical Operator2/1 -> 高电平计数/1
  Data Type Conversion4/1 -> 高电平计数/2
  Switch3/1 -> aL1/1

== system yixiang/CBSVPWM/jxcbsv/yixiang5/zmc1 ==
  aH1 : Inport
  Constant2 : Constant  OutDataTypeStr=int16  SampleTime=2E-8
  Constant3 : Constant  Commented=on  Value=0  OutDataTypeStr=int16  SampleTime=2e-8
  Data Type Conversion1 : DataTypeConversion  OutDataTypeStr=boolean  SaturateOnIntegerOverflow=off  RndMeth=Floor
  Data Type Conversion2 : DataTypeConversion  OutDataTypeStr=boolean  SaturateOnIntegerOverflow=off  RndMeth=Floor
  Data Type Conversion3 : DataTypeConversion  Commented=on  OutDataTypeStr=boolean  SaturateOnIntegerOverflow=off  RndMeth=Floor
  HDL Counter1 : hdlsllib/Sources/HDL Counter  Commented=on  CountType=Free running  CountInit=0  CountStep=1  CountMax=250  CountFromType=Initial value  CountFrom=0  CountResetPort=on  CountLoadPort=off  CountEnbPort=off  CountDirPort=off  CountHitOutputPort=off  CountDataType=Signed  CountWordLen=16  CountFracLen=0  CountSampTime=2E-8
  HDL Counter7 : hdlsllib/Sources/HDL Counter  CountType=Free running  CountInit=0  CountStep=1  CountMax=250  CountFromType=Initial value  CountFrom=0  CountResetPort=on  CountLoadPort=off  CountEnbPort=on  CountDirPort=off  CountHitOutputPort=off  CountDataType=Signed  CountWordLen=16  CountFracLen=0  CountSampTime=1
  Logical Operator : Logic  Operator=NOT  AllPortsSameDT=off  OutDataTypeStr=boolean
  Logical Operator1 : Logic  Commented=on  Operator=NOT  AllPortsSameDT=off  OutDataTypeStr=boolean
  Scope6 : Scope  NumInputPorts=2
  Switch : Switch  Threshold=3  SaturateOnIntegerOverflow=off  InputSameDT=off
  Switch2 : Switch  Commented=on  Threshold=1  SaturateOnIntegerOverflow=off  InputSameDT=off
  bH1 : Outport
  wires:
  HDL Counter7/1 -> Switch/2, Scope6/1
  Data Type Conversion1/1 -> Logical Operator/1
  Constant2/1 -> Switch/3
  aH1/1 -> Data Type Conversion1/1, Scope6/2, Data Type Conversion2/1, Switch/1
  Logical Operator/1 -> HDL Counter7/2
  Data Type Conversion2/1 -> HDL Counter7/1
  Constant3/1 -> Switch2/3
  HDL Counter1/1 -> Switch2/2
  Switch/1 -> bH1/1
  Data Type Conversion3/1 -> Logical Operator1/1
  Logical Operator1/1 -> HDL Counter1/1

== system yixiang/CBSVPWM/jxcbsv/yixiang5/zmcxc6 ==
  bH1 : Inport
  Constant2 : Constant  Value=0  OutDataTypeStr=int16  SampleTime=2e-8
  Data Type Conversion3 : DataTypeConversion  OutDataTypeStr=boolean  SaturateOnIntegerOverflow=off  RndMeth=Floor
  Data Type Conversion4 : DataTypeConversion  OutDataTypeStr=boolean  SaturateOnIntegerOverflow=off  RndMeth=Floor
  Logical Operator2 : Logic  Operator=NOT  AllPortsSameDT=off  OutDataTypeStr=boolean
  Switch3 : Switch  Threshold=6  SaturateOnIntegerOverflow=off  InputSameDT=off
  高电平计数 : hdlsllib/Sources/HDL Counter  CountType=Free running  CountInit=0  CountStep=1  CountMax=250  CountFromType=Initial value  CountFrom=0  CountResetPort=on  CountLoadPort=off  CountEnbPort=on  CountDirPort=off  CountHitOutputPort=off  CountDataType=Signed  CountWordLen=16  CountFracLen=0  CountSampTime=1
  aL1 : Outport
  wires:
  Data Type Conversion3/1 -> Logical Operator2/1
  bH1/1 -> Switch3/1, Data Type Conversion4/1, Data Type Conversion3/1
  Constant2/1 -> Switch3/3
  高电平计数/1 -> Switch3/2
  Logical Operator2/1 -> 高电平计数/1
  Data Type Conversion4/1 -> 高电平计数/2
  Switch3/1 -> aL1/1

== system yixiang/CBSVPWM/jxcbsv/yixianga/zmc1 ==
  aH1 : Inport
  Constant2 : Constant  OutDataTypeStr=int16  SampleTime=2E-8
  Constant3 : Constant  Commented=on  Value=0  OutDataTypeStr=int16  SampleTime=2e-8
  Data Type Conversion1 : DataTypeConversion  OutDataTypeStr=boolean  SaturateOnIntegerOverflow=off  RndMeth=Floor
  Data Type Conversion2 : DataTypeConversion  OutDataTypeStr=boolean  SaturateOnIntegerOverflow=off  RndMeth=Floor
  Data Type Conversion3 : DataTypeConversion  Commented=on  OutDataTypeStr=boolean  SaturateOnIntegerOverflow=off  RndMeth=Floor
  HDL Counter1 : hdlsllib/Sources/HDL Counter  Commented=on  CountType=Free running  CountInit=0  CountStep=1  CountMax=250  CountFromType=Initial value  CountFrom=0  CountResetPort=on  CountLoadPort=off  CountEnbPort=off  CountDirPort=off  CountHitOutputPort=off  CountDataType=Signed  CountWordLen=16  CountFracLen=0  CountSampTime=2E-8
  HDL Counter7 : hdlsllib/Sources/HDL Counter  CountType=Free running  CountInit=0  CountStep=1  CountMax=250  CountFromType=Initial value  CountFrom=0  CountResetPort=on  CountLoadPort=off  CountEnbPort=on  CountDirPort=off  CountHitOutputPort=off  CountDataType=Signed  CountWordLen=16  CountFracLen=0  CountSampTime=1
  Logical Operator : Logic  Operator=NOT  AllPortsSameDT=off  OutDataTypeStr=boolean
  Logical Operator1 : Logic  Commented=on  Operator=NOT  AllPortsSameDT=off  OutDataTypeStr=boolean
  Scope6 : Scope  NumInputPorts=2
  Switch : Switch  Threshold=3  SaturateOnIntegerOverflow=off  InputSameDT=off
  Switch2 : Switch  Commented=on  Threshold=1  SaturateOnIntegerOverflow=off  InputSameDT=off
  bH1 : Outport
  wires:
  HDL Counter7/1 -> Switch/2, Scope6/1
  Data Type Conversion1/1 -> Logical Operator/1
  Constant2/1 -> Switch/3
  aH1/1 -> Data Type Conversion1/1, Scope6/2, Data Type Conversion2/1, Switch/1
  Logical Operator/1 -> HDL Counter7/2
  Data Type Conversion2/1 -> HDL Counter7/1
  Constant3/1 -> Switch2/3
  HDL Counter1/1 -> Switch2/2
  Switch/1 -> bH1/1
  Data Type Conversion3/1 -> Logical Operator1/1
  Logical Operator1/1 -> HDL Counter1/1

== system yixiang/CBSVPWM/jxcbsv/yixianga/zmcxc6 ==
  bH1 : Inport
  Constant2 : Constant  Value=0  OutDataTypeStr=int16  SampleTime=2e-8
  Data Type Conversion3 : DataTypeConversion  OutDataTypeStr=boolean  SaturateOnIntegerOverflow=off  RndMeth=Floor
  Data Type Conversion4 : DataTypeConversion  OutDataTypeStr=boolean  SaturateOnIntegerOverflow=off  RndMeth=Floor
  Logical Operator2 : Logic  Operator=NOT  AllPortsSameDT=off  OutDataTypeStr=boolean
  Switch3 : Switch  Threshold=6  SaturateOnIntegerOverflow=off  InputSameDT=off
  高电平计数 : hdlsllib/Sources/HDL Counter  CountType=Free running  CountInit=0  CountStep=1  CountMax=250  CountFromType=Initial value  CountFrom=0  CountResetPort=on  CountLoadPort=off  CountEnbPort=on  CountDirPort=off  CountHitOutputPort=off  CountDataType=Signed  CountWordLen=16  CountFracLen=0  CountSampTime=1
  aL1 : Outport
  wires:
  Data Type Conversion3/1 -> Logical Operator2/1
  bH1/1 -> Switch3/1, Data Type Conversion4/1, Data Type Conversion3/1
  Constant2/1 -> Switch3/3
  高电平计数/1 -> Switch3/2
  Logical Operator2/1 -> 高电平计数/1
  Data Type Conversion4/1 -> 高电平计数/2
  Switch3/1 -> aL1/1
